simulink model "s_bb01_pos"  (R2021b)
settings: Solver=ode4  StartTime=0.0  StopTime=25  FixedStep=0.002  RelTol=1e-3  AbsTol=1e-6  EnableMultiTasking=on
values from neighbouring files (symbols this model uses):
  K = Am / Beq_v    [d_model_param.m]
  K_AMP = 1    [setup_srv02_exp04_bb01.m]
  K_bb = m_b * g * r_arm / L_beam * r_b^2 / ( m_b * r_b^2 + J_b )    [d_bb01_model_param.m]    (also in setup_srv02_exp04_bb01.m = 0)
  Kc = wn^2 / (Tp*K_bb*z*wf)    [d_bb01_pd.m]    (also in setup_srv02_exp04_bb01.m = 0)
  kp = (wn^2/K)*tau    [d_pv_design.m]    (also in setup_srv02_exp04_bb01.m = 0)
  kv = (-1+2*zeta*wn*tau)/K    [d_pv_design.m]    (also in setup_srv02_exp04_bb01.m = 0)
  tau = Jeq / Beq_v    [d_model_param.m]
  THETA_MAX = 56.0 * K_D2R    [config_bb01.m]
  THETA_MIN = - 56.0 * K_D2R    [config_bb01.m]
  VMAX_DAC = 10    [setup_srv02_exp04_bb01.m]
  wcf = 2 * pi * 50.0    (= 314.159265359)    [setup_srv02_exp04_bb01.m]
  wf = 2 * pi * 2.5    (= 15.7079632679)    [d_bb01_pd.m]    (also in setup_srv02_exp04_bb01.m = 6.28318530718)
  z = wn*wf/(-wn+wf*wn*Tp+2*wf*zeta)    [d_bb01_pd.m]    (also in setup_srv02_exp04_bb01.m = 1)
  zetaf = 0.9    [setup_srv02_exp04_bb01.m]
undefined symbols (not defined in the file or in its folder): VMAX_AMP
libraries: simulink x3, simulink_extras x1
settings Model: ExtModeTrigDuration=10000  Creator=MLevis  LastModifiedBy=Dell
settings SolverCC: AutoScaleAbsTol=off  AlgebraicLoopSolver=TrustRegion  PositivePriorityOrder=on
settings DataIOCC: SaveFormat=Array  SignalLoggingSaveFormat=ModelDataLogs  ReturnWorkspaceOutputs=off
settings OptimizationCC: BlockReduction=off  BooleanDataType=off  OptimizeBlockIOStorage=off  BufferReuse=off  ExpressionFolding=off  ExpressionDepthLimit=2147483647  LocalBlockOutputs=off  InitFltsAndDblsToZero=on
settings DebuggingCC: SaveWithParameterizedLinksMsg=none  UnderspecifiedInitializationDetection=Classic  MergeDetectMultiDrivingBlocksExec=none  SignalResolutionControl=TryResolveAllWithWarning  MultiTaskDSMMsg=warning  MultiTaskCondExecSysMsg=none  FcnCallInpInsideContextMsg=warning  StateNameClashWarn=warning  SFUnexpectedBacktrackingDiag=warning  SFNoUnconditionalDefaultTransitionDiag=warning  SFExecutionAtInitializationDiag=none  SFMachineParentedDataDiag=warning  ArithmeticOperatorsInVariantConditions=warning
settings HardwareCC: TargetHWDeviceType=32-bit Generic
settings ModelReferenceCC: PropagateSignalLabelsOutOfModel=off
settings RTWCC: Description=QUARC Win64 Target Using Toolchain  SystemTargetFile=quarc_win64.tlc  TemplateMakefile=quarc_default_tmf  Toolchain=QUARC win64 | nmake (64-bit Windows)  BuildConfiguration=Faster Runs
settings CodeAppCC: StateflowObjectComments=on
settings STFCustomTargetCC: ConcurrentExecutionCompliant=on  UseToolchainInfoCompliant=on  SystemTargetFile=quarc_win64.tlc
settings GRTTargetCC: TargetLangStandard=C89/C90 (ANSI)  ParMdlRefBuildCompliant=off  CompOptLevelCompliant=off  CombineOutputUpdateFcns=off  MatFileLogging=off  CPPClassGenCompliant=off  GRTInterface=on  ExtMode=on  ExtModeMexFile=quarc_comm
settings ConfigComp: CovMetricSettings=dw  CovSaveCumulativeToWorkspaceVar=on  CovSaveSingleToWorkspaceVar=on

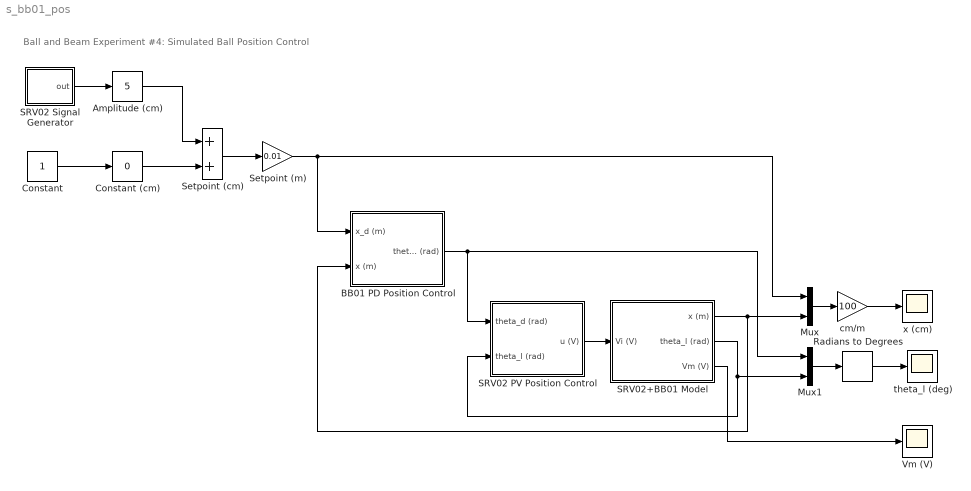
== system s_bb01_pos ==
  note: Ball and Beam Experiment #4: Simulated Ball Position Control
  Amplitude (cm) : simulink/Math Operations/Slider Gain  gain=5  low=-10  high=10
  BB01 PD Position Control : Subsystem
  "Constant " : Constant
  Constant (cm) : simulink/Math Operations/Slider Gain  gain=0  low=-20  high=20
  Mux : Mux  Inputs=2
  Mux1 : Mux  Inputs=2
  Radians to Degrees : simulink_extras/Transformations/Radians to Degrees
  SRV02 PV Position Control : Subsystem
  SRV02 Signal Generator : Subsystem  mask(QET Signal Generator){sig_type=square, a=1, f=0.05}
      mask prompts: sig_type "Signal Type"; a "Amplitude"; f "Frequency (Hz)"
      mask help: Generates a square, triangular, or sinusoidal waveform of a specified amplitude and frequency.
      mask Help: Choose the type of signal to be generated from the drop-down "Signal Type" box. Enter the amplitude and the frequency desired for the signal. Note: frequency is in Hertz.
      mask TypeOptions sig_type: square | triangle | sine
      mask Display: plot([0 1 1 2 2 3 4 5 6], [-1 -1 1 1 -1 -1 1 -1 -1])
  SRV02+BB01 Model : Subsystem
  Setpoint (cm) : Sum
  Setpoint (m) : Gain  Gain=0.01
  Vm (V) : Scope
  cm/m : Gain  Gain=100
  theta_l (deg) : Scope
  x (cm) : Scope
  wires:
  Mux/1 -> cm/m/1
  SRV02 PV Position Control/1(u (V)) -> SRV02+BB01 Model/1(Vi (V))
  SRV02 Signal Generator/1(out) -> Amplitude (cm)/1
  Constant (cm)/1 -> Setpoint (cm)/2
  "Constant "/1 -> Constant (cm)/1
  Amplitude (cm)/1 -> Setpoint (cm)/1
  Setpoint (cm)/1 -> Setpoint (m)/1
  SRV02+BB01 Model/2(theta_l (rad)) -> SRV02 PV Position Control/2(theta_l (rad)), Mux1/2
  SRV02+BB01 Model/1(x (m)) -> Mux/2, BB01 PD Position Control/2(x (m))
  SRV02+BB01 Model/3(Vm (V)) -> Vm (V)/1
  Mux1/1 -> Radians to Degrees/1
  Setpoint (m)/1 -> Mux/1, BB01 PD Position Control/1(x_d (m))
  Radians to Degrees/1 -> theta_l (deg)/1
  cm/m/1 -> x (cm)/1
  BB01 PD Position Control/1(theta_d (rad)) -> SRV02 PV Position Control/1(theta_d (rad)), Mux1/1

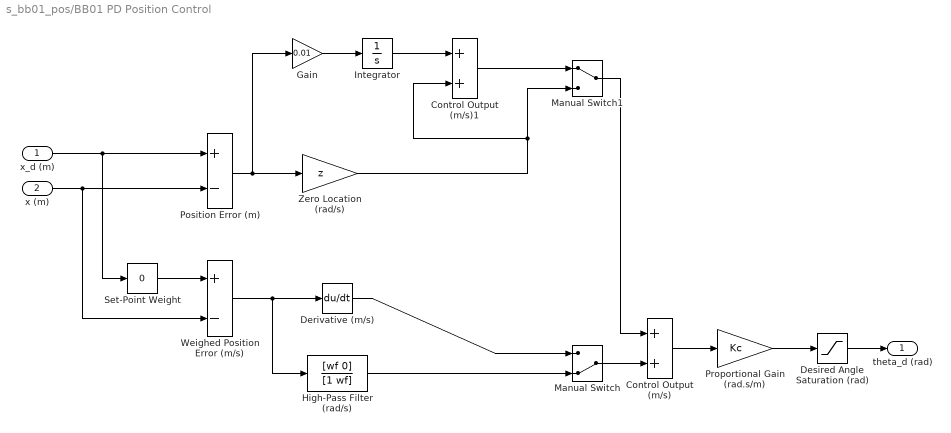
== system s_bb01_pos/BB01 PD Position Control ==
  x_d (m) : Inport
  x (m) : Inport  Port=2
  Control Output (m/s) : Sum
  Control Output (m/s)1 : Sum
  Derivative (m/s) : Derivative
  Desired Angle Saturation (rad) : Saturate  UpperLimit=THETA_MAX  LowerLimit=THETA_MIN
  Gain : Gain  Gain=0.01
  High-Pass Filter (rad/s) : TransferFcn  Numerator=[wf 0]  Denominator=[1 wf]
  Integrator : Integrator
  Manual Switch : ManualSwitch  CurrentSetting=0
  Manual Switch1 : ManualSwitch
  Position Error (m) : Sum  Inputs=+-
  Proportional Gain (rad.s/m) : Gain  Gain=Kc
  Set-Point Weight : simulink/Math Operations/Slider Gain  gain=0  low=0  high=1
  Weighed Position Error (m/s) : Sum  Inputs=+-
  Zero Location (rad/s) : Gain  Gain=z
  theta_d (rad) : Outport
  wires:
  Zero Location (rad/s)/1 -> Manual Switch1/2, Control Output (m/s)1/2
  Position Error (m)/1 -> Gain/1, Zero Location (rad/s)/1
  Weighed Position Error (m/s)/1 -> Derivative (m/s)/1, High-Pass Filter (rad/s)/1
  Set-Point Weight/1 -> Weighed Position Error (m/s)/1
  Proportional Gain (rad.s/m)/1 -> Desired Angle Saturation (rad)/1
  Control Output (m/s)/1 -> Proportional Gain (rad.s/m)/1
  x_d (m)/1 -> Set-Point Weight/1, Position Error (m)/1
  x (m)/1 -> Weighed Position Error (m/s)/2, Position Error (m)/2
  Desired Angle Saturation (rad)/1 -> theta_d (rad)/1
  Derivative (m/s)/1 -> Manual Switch/1
  High-Pass Filter (rad/s)/1 -> Manual Switch/2
  Manual Switch/1 -> Control Output (m/s)/2
  Manual Switch1/1 -> Control Output (m/s)/1
  Integrator/1 -> Control Output (m/s)1/1
  Control Output (m/s)1/1 -> Manual Switch1/1
  Gain/1 -> Integrator/1

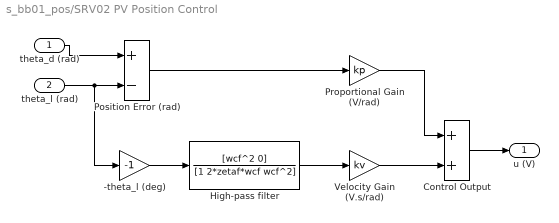
== system s_bb01_pos/SRV02 PV Position Control ==
  theta_d (rad) : Inport
  theta_l (rad) : Inport  Port=2
  -theta_l (deg) : Gain  Gain=-1
  Control Output : Sum
  High-pass filter : TransferFcn  Numerator=[wcf^2 0]  Denominator=[1 2*zetaf*wcf wcf^2]
  Position Error (rad) : Sum  Inputs=+-
  Proportional Gain (V/rad) : Gain  Gain=kp
  Velocity Gain (V.s/rad) : Gain  Gain=kv
  u (V) : Outport
  wires:
  Proportional Gain (V/rad)/1 -> Control Output/1
  theta_d (rad)/1 -> Position Error (rad)/1
  Control Output/1 -> u (V)/1
  theta_l (rad)/1 -> Position Error (rad)/2, -theta_l (deg)/1
  Position Error (rad)/1 -> Proportional Gain (V/rad)/1
  Velocity Gain (V.s/rad)/1 -> Control Output/2
  -theta_l (deg)/1 -> High-pass filter/1
  High-pass filter/1 -> Velocity Gain (V.s/rad)/1

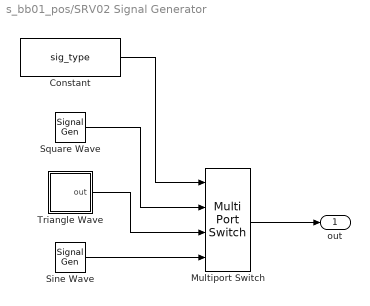
== system s_bb01_pos/SRV02 Signal Generator ==
  Constant : Constant  Value=sig_type
  Multiport Switch : MultiPortSwitch
  Sine Wave : SignalGenerator  Amplitude=a  Frequency=f
  Square Wave : SignalGenerator  WaveForm=square  Amplitude=a  Frequency=f
  Triangle Wave : Subsystem
  out : Outport
  wires:
  Square Wave/1 -> Multiport Switch/2
  Triangle Wave/1(out) -> Multiport Switch/3
  Sine Wave/1 -> Multiport Switch/4
  Multiport Switch/1 -> out/1
  Constant/1 -> Multiport Switch/1

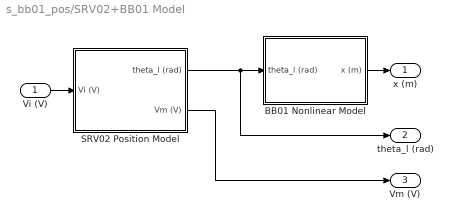
== system s_bb01_pos/SRV02+BB01 Model ==
  Vi (V) : Inport
  BB01 Nonlinear Model : Subsystem
  SRV02 Position Model : Subsystem
  x (m) : Outport
  theta_l (rad) : Outport  Port=2
  Vm (V) : Outport  Port=3
  wires:
  SRV02 Position Model/1(theta_l (rad)) -> BB01 Nonlinear Model/1(theta_l (rad)), theta_l (rad)/1
  BB01 Nonlinear Model/1(x (m)) -> x (m)/1
  Vi (V)/1 -> SRV02 Position Model/1(Vi (V))
  SRV02 Position Model/2(Vm (V)) -> Vm (V)/1

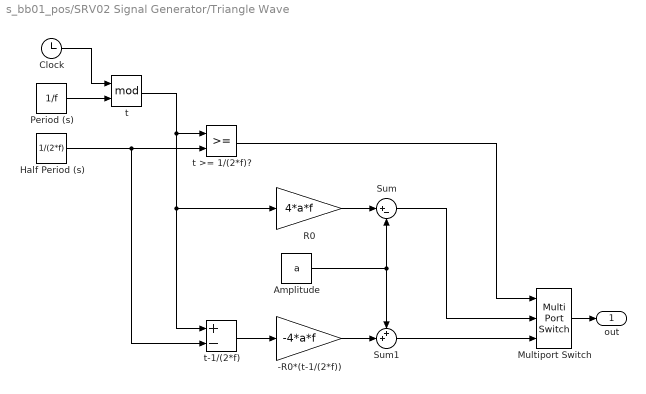
== system s_bb01_pos/SRV02 Signal Generator/Triangle Wave ==
  -R0*(t-1/(2*f)) : Gain  Gain=-4*a*f
  Amplitude : Constant  Value=a
  Clock : Clock
  Half Period (s) : Constant  Value=1/(2*f)
  Multiport Switch : MultiPortSwitch  DataPortOrder=Zero-based contiguous  Inputs=2  zeroidx=on
  Period (s) : Constant  Value=1/f
  R0 : Gain  Gain=4*a*f
  Sum : Sum  Inputs=|+-
  Sum1 : Sum  Inputs=++|
  t : Math  Operator=mod  SignedPower=on  SaturateOnIntegerOverflow=on
  t >= 1/(2*f)? : RelationalOperator  OutDataTypeStr=boolean  RndMeth=Nearest
  t-1/(2*f) : Sum  Inputs=+-
  out : Outport
  wires:
  Sum1/1 -> Multiport Switch/3
  Sum/1 -> Multiport Switch/2
  t >= 1/(2*f)?/1 -> Multiport Switch/1
  -R0*(t-1/(2*f))/1 -> Sum1/2
  Amplitude/1 -> Sum1/1, Sum/2
  R0/1 -> Sum/1
  t-1/(2*f)/1 -> -R0*(t-1/(2*f))/1
  Half Period (s)/1 -> t-1/(2*f)/2, t >= 1/(2*f)?/2
  t/1 -> t-1/(2*f)/1, R0/1, t >= 1/(2*f)?/1
  Period (s)/1 -> t/2
  Clock/1 -> t/1
  Multiport Switch/1 -> out/1

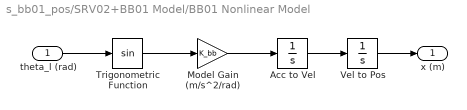
== system s_bb01_pos/SRV02+BB01 Model/BB01 Nonlinear Model ==
  theta_l (rad) : Inport
  Acc to Vel : Integrator
  Model Gain (m/s^2/rad) : Gain  Gain=K_bb
  Trigonometric Function : Trigonometry
  Vel to Pos : Integrator
  x (m) : Outport
  wires:
  theta_l (rad)/1 -> Trigonometric Function/1
  Vel to Pos/1 -> x (m)/1
  Model Gain (m/s^2/rad)/1 -> Acc to Vel/1
  Acc to Vel/1 -> Vel to Pos/1
  Trigonometric Function/1 -> Model Gain (m/s^2/rad)/1

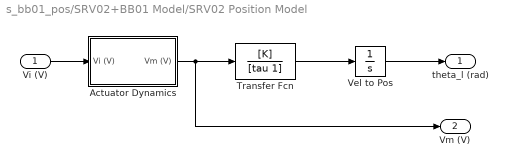
== system s_bb01_pos/SRV02+BB01 Model/SRV02 Position Model ==
  Vi (V) : Inport
  Actuator Dynamics : Subsystem
  Transfer Fcn : TransferFcn  Numerator=[K]  Denominator=[tau 1]
  Vel to Pos : Integrator
  theta_l (rad) : Outport
  Vm (V) : Outport  Port=2
  wires:
  Transfer Fcn/1 -> Vel to Pos/1
  Vel to Pos/1 -> theta_l (rad)/1
  Actuator Dynamics/1(Vm (V)) -> Transfer Fcn/1, Vm (V)/1
  Vi (V)/1 -> Actuator Dynamics/1(Vi (V))

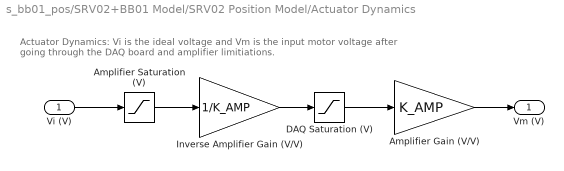
== system s_bb01_pos/SRV02+BB01 Model/SRV02 Position Model/Actuator Dynamics ==
  note: Actuator Dynamics: Vi is the ideal voltage and Vm is the
      | input motor voltage after going through the DAQ board and amplifier limitiations.
  Vi (V) : Inport
  Amplifier Gain (V/V) : Gain  Gain=K_AMP
  Amplifier Saturation (V) : Saturate  UpperLimit=VMAX_AMP  LowerLimit=-VMAX_AMP
  DAQ Saturation (V) : Saturate  UpperLimit=VMAX_DAC  LowerLimit=-VMAX_DAC
  Inverse Amplifier Gain (V/V) : Gain  Gain=1/K_AMP
  Vm (V) : Outport
  wires:
  DAQ Saturation (V)/1 -> Amplifier Gain (V/V)/1
  Inverse Amplifier Gain (V/V)/1 -> DAQ Saturation (V)/1
  Amplifier Gain (V/V)/1 -> Vm (V)/1
  Vi (V)/1 -> Amplifier Saturation (V)/1
  Amplifier Saturation (V)/1 -> Inverse Amplifier Gain (V/V)/1
